simulink model "AFO_Assistance"  (R2024a)
settings: Solver=FixedStepAuto  StartTime=0.0  StopTime=inf  FixedStep=0.001  RelTol=1e-3  EnableMultiTasking=on
libraries: slrealtimeethercatlib x15, simulink_extras x5, simulink x1, slpidlib x1
(part 1 of 2)
settings Model: SimulationMode=external  ExtModeEnableFloating=off  Creator=mbout  LastModifiedBy=Andy
settings SolverCC: ConcurrentTasks=on  AlgebraicLoopSolver=TrustRegion  PositivePriorityOrder=on  AutoInsertRateTranBlk=on  InsertRTBMode=Never (minimum delay)
settings DataIOCC: SaveFormat=Array  SaveState=on  SignalLoggingName=logsOut
settings OptimizationCC: BlockReduction=off  BooleanDataType=off  OptimizeBlockIOStorage=off  BufferReuse=off  ReuseModelBlockBuffer=off  GlobalBufferReuse=off  ExpressionFolding=off  LocalBlockOutputs=off  InitFltsAndDblsToZero=on  OptimizeDataStoreBuffers=off  BusAssignmentInplaceUpdate=off
settings DebuggingCC: SaveWithParameterizedLinksMsg=none  UnderspecifiedInitializationDetection=Classic  MergeDetectMultiDrivingBlocksExec=none  CheckExecutionContextPreStartOutputMsg=on  SignalResolutionControl=TryResolveAllWithWarning  TasksWithSamePriorityMsg=none  ParameterPrecisionLossMsg=none  UnconnectedInputMsg=warning  UnconnectedOutputMsg=warning  UnconnectedLineMsg=warning  SFUnexpectedBacktrackingDiag=warning  SFNoUnconditionalDefaultTransitionDiag=warning  SFExecutionAtInitializationDiag=none  ArithmeticOperatorsInVariantConditions=warning
settings HardwareCC: ProdBitPerLong=64  ProdLongLongMode=on  ProdHWDeviceType=Intel->x86-64 (Linux 64)
settings ModelReferenceCC: EnableRefExpFcnMdlSchedulingChecks=on  PropagateSignalLabelsOutOfModel=off
settings SFSimCC: SimUseLocalCustomCode=off  SimTargetLang=C++
settings RTWCC: Description=Speedgoat Real-Time Target Machine  SystemTargetFile=speedgoat.tlc  TemplateMakefile=slrealtime_default_tmf  RTWUseLocalCustomCode=off  Toolchain=Simulink Real-Time Toolchain  BuildConfiguration=Faster Runs  CodeExecutionProfiling=on  TargetLang=C++  GPUComputeCapability=3.5  DLArmComputeVersion=19.05
settings CodeAppCC: StateflowObjectComments=on
settings SimulinkRealTimeTargetCC: InstructionSetFMA=off  LogToMDFFile=off
settings ConfigComp: CovMetricSettings=dw  CovSaveCumulativeToWorkspaceVar=on  CovSaveSingleToWorkspaceVar=on  CovExternalEMLEnable=off  CovSFcnEnable=off

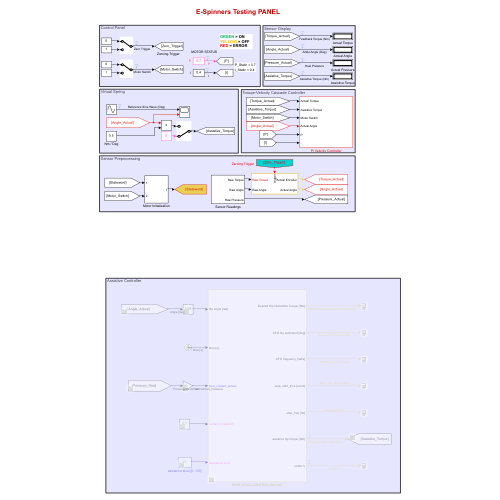
[thumbnail: Simulink's stored preview of the top-level diagram]
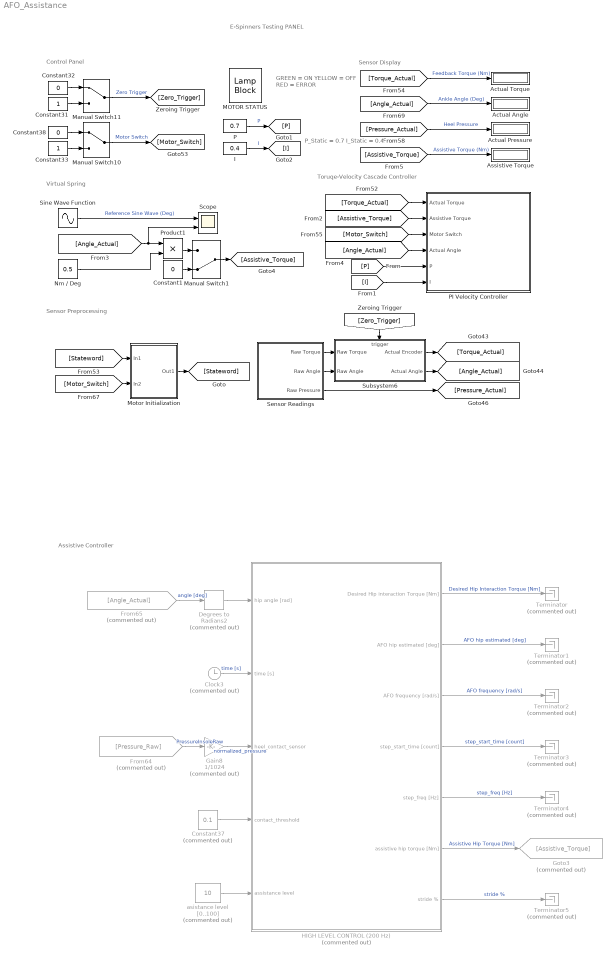
== system AFO_Assistance ==
  note: Sensor Display
  note: E-Spinners Testing PANEL
  note: GREEN = ON
      | YELLOW = OFF
      | RED = ERROR
  note: Control Panel
  note: Toruqe-Velocity Cascade Controller
  note: Sensor Preprocessing
  note: P_Static = 0.7
      | I_Static = 0.4
  note: Assistive Controller
  note: Virtual Spring
  Actual Angle : Display
  Actual Pressure : Display
  Actual Torque : Display
  Assistive Torque : Display
  Clock3 : Clock  Commented=on
  Constant1 : Constant  Value=0
  Constant31 : Constant
  Constant32 : Constant  Value=0
  Constant33 : Constant
  Constant37 : Constant  Commented=on  Value=0.1
  Constant38 : Constant  Value=0
  Degrees to Radians2 : simulink_extras/Transformations/Degrees to Radians  Commented=on
  From64 : From  Commented=on  GotoTag=Pressure_Raw
  From65 : From  Commented=on  GotoTag=Angle_Actual
  Gain8 : Gain  Commented=on  Gain=1/1024
  Goto3 : Goto  Commented=on  GotoTag=Assistive_Torque
  HIGH LEVEL CONTROL (200 Hz) : Subsystem  Commented=on
  I : Constant  Value=0.4
  MOTOR STATUS : LampBlock  LabelPosition=Hide
  Manual Switch1 : ManualSwitch  CurrentSetting=0
  Manual Switch10 : ManualSwitch
  Manual Switch11 : ManualSwitch
  Motor Initialization : Subsystem
  Nm / Deg : Constant  Value=0.5
  P : Constant  Value=0.7
  PI Velocity Controller : Subsystem
  Product1 : Product
  Scope : Scope  NumInputPorts=2
  Sensor Readings : Subsystem
  Sine Wave Function : Sin  Amplitude=24  Frequency=0.5 * 6.28  SampleTime=0
  Subsystem6 : Subsystem  TreatAsAtomicUnit=on
      settings: PortSchema="{\"entries\":[{\"content\":{\"sides\":[{\"content\":{\"connectorIds\":[\"In1\",\"In2\"]},\"type\":\"ConnectorPlacement.EquallySpacedRectSide\",\"uuid\":\"9f3d9f1a-9a54-41ee-920c-c2d0f371d202\"},{\"content\":{\"connectorIds\":[\"Out1\",\"Out2\"],\"side\":\"RIGHT\"},\"type\":\"ConnectorPlacement.EquallySpacedRectSide\",\"uuid\":\"1f39d886-5c2a-4ad9-bf33-c1da713dba43\"},{\"content\":{\"connectorIds\":[\"In3\"],\"side\":\"TOP\"},\"type\":\"ConnectorPlacement.EquallySpacedRectSide\",\"uuid\":\"f96becb7-64eb-4482-a661-ce8cddc3e5ff\"}]},\"type\":\"ConnectorPlacement.EquallySpacedConnector\",\"uuid\":\"ca43ddc1-706b-467a-b9cf-4d299dd568f6\"}],\"packageUris\":[\"http://schema.mathworks.com/mf0/Connector/R2020b\"],\"version\":\"1.0\"}"
  Terminator{,1..5} (6 alike) : Terminator  Commented=on
  asistance level [0..100] : Constant  Commented=on  Value=10  OutMin=[0]  OutMax=[100]  SampleTime=0.01
  wires:
  [Torque_Actual] -> Actual Torque/1  "Feedback Torque (Nm)"
  [Angle_Actual] -> Actual Angle/1  "Ankle Angle (Deg)"
  [Zero_Trigger] -> Subsystem6/3(trigger)
  Subsystem6/2(Actual Angle) -> [Angle_Actual]
  HIGH LEVEL CONTROL (200 Hz)/4(step_start_time [count]) -> Terminator3/1  "step_start_time [count]"
  HIGH LEVEL CONTROL (200 Hz)/7(stride %) -> Terminator5/1  "stride %"
  HIGH LEVEL CONTROL (200 Hz)/3(AFO frequency [rad/s]) -> Terminator2/1  "AFO frequency [rad/s]"
  From64/1 -> Gain8/1  "PressureInsoleRaw"
  Constant32/1 -> Manual Switch11/1
  Subsystem6/1(Actual Encoder) -> [Torque_Actual]
  Degrees to Radians2/1 -> HIGH LEVEL CONTROL (200 Hz)/1(hip angle [rad])
  [Pressure_Actual] -> Actual Pressure/1  "Heel Pressure"
  Gain8/1 -> HIGH LEVEL CONTROL (200 Hz)/3(heel_contact_sensor)  "normalized_pressure"
  HIGH LEVEL CONTROL (200 Hz)/2(AFO hip estimated [deg]) -> Terminator1/1  "AFO hip estimated [deg]"
  From65/1 -> Degrees to Radians2/1  "angle [deg]"
  [Torque_Actual] -> PI Velocity Controller/1(Actual Torque)
  HIGH LEVEL CONTROL (200 Hz)/1(Desired Hip interaction Torque [Nm]) -> Terminator/1  "Desired Hip Interaction Torque [Nm]"
  [I] -> PI Velocity Controller/6(I)
  Constant37/1 -> HIGH LEVEL CONTROL (200 Hz)/4(contact_threshold)
  Constant31/1 -> Manual Switch11/2
  Constant33/1 -> Manual Switch10/2
  [Motor_Switch] -> PI Velocity Controller/3(Motor Switch)
  Constant38/1 -> Manual Switch10/1
  Manual Switch10/1 -> [Motor_Switch]  "Motor Switch"
  [P] -> PI Velocity Controller/5(P)
  Sensor Readings/2(Raw Angle) -> Subsystem6/2(Raw Angle)
  Manual Switch11/1 -> [Zero_Trigger]  "Zero Trigger"
  HIGH LEVEL CONTROL (200 Hz)/6(assistive hip torque [Nm]) -> Goto3/1  "Assistive Hip Torque [Nm]"
  Clock3/1 -> HIGH LEVEL CONTROL (200 Hz)/2(time [s])  "time [s]"
  HIGH LEVEL CONTROL (200 Hz)/5(step_freq [Hz]) -> Terminator4/1  "step_freq [Hz]"
  P/1 -> [P]  "P"
  I/1 -> [I]  "I"
  [Assistive_Torque] -> PI Velocity Controller/2(Assistive Torque)
  [Angle_Actual] -> Product1/1, Scope/2
  Nm / Deg/1 -> Product1/2
  Sine Wave Function/1 -> Scope/1  "Reference Sine Wave (Deg)"
  Manual Switch1/1 -> [Assistive_Torque]
  asistance level [0..100]/1 -> HIGH LEVEL CONTROL (200 Hz)/5(assistance level)
  [Stateword] -> Motor Initialization/1(In1)
  [Motor_Switch] -> Motor Initialization/2(In2)
  Motor Initialization/1(Out1) -> [Stateword]
  Product1/1 -> Manual Switch1/1
  Constant1/1 -> Manual Switch1/2
  [Angle_Actual] -> PI Velocity Controller/4(Actual Angle)
  Sensor Readings/3(Raw Pressure) -> [Pressure_Actual]
  Sensor Readings/1(Raw Torque) -> Subsystem6/1(Raw Torque)
  [Assistive_Torque] -> Assistive Torque/1  "Assistive Torque (Nm)"

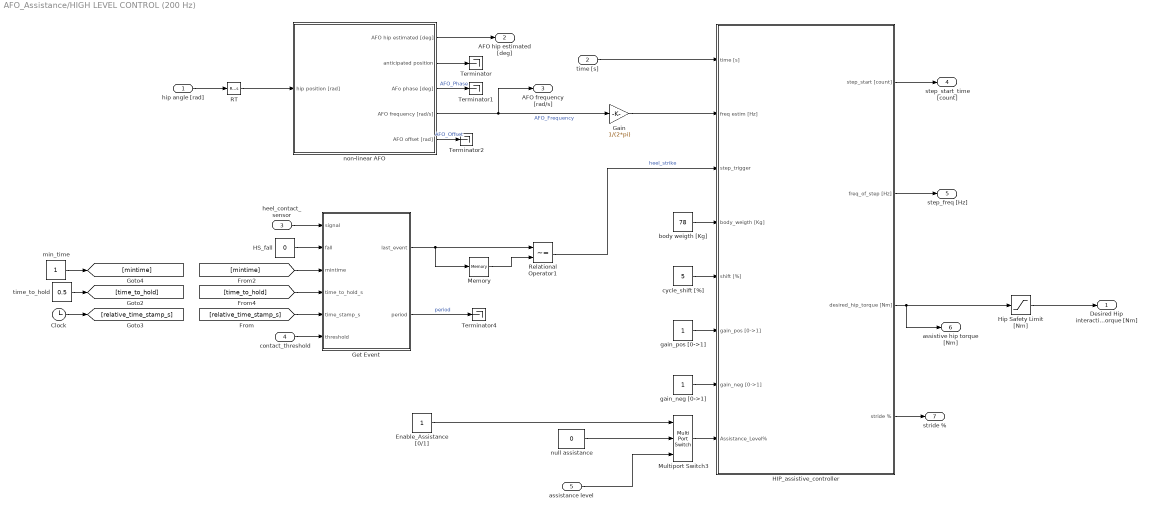
== system AFO_Assistance/HIGH LEVEL CONTROL (200 Hz) ==
  hip angle [rad] : Inport
  time [s] : Inport  Port=2
  heel_contact_sensor : Inport  Port=3
  contact_threshold : Inport  Port=4
  assistance level : Inport  Port=5
  Clock : Clock
  Enable_Assistance [0/1] : Constant  OutMin=[0]  OutMax=[1]  SampleTime=0.01
  Gain : Gain  Gain=1/(2*pi)
  Get Event : Subsystem  TreatAsAtomicUnit=on  SystemSampleTime=1/200
  HIP_assistive_controller : Subsystem
  HS_fall : Constant  Value=0
  Hip Safety Limit [Nm] : Saturate  UpperLimit=50  LowerLimit=-50  SampleTime=0.01
  Memory : Memory
  Multiport Switch3 : MultiPortSwitch  DataPortOrder=Zero-based contiguous  Inputs=2  zeroidx=on  SampleTime=0.01  SaturateOnIntegerOverflow=off  InputSameDT=off
  RT : RateTransition  Deterministic=off  OutPortSampleTime=1/200
  Relational Operator1 : RelationalOperator  Operator=~=  OutDataTypeStr=boolean  RndMeth=Simplest  InputSameDT=off
  Terminator{,1..2,4} (4 alike) : Terminator
  body weigth [Kg] : Constant  Value=78  OutMin=[0]  OutMax=[100]  SampleTime=0.01
  cycle_shift [%] : Constant  Value=5  OutMin=[0]  OutMax=[20]  SampleTime=0.01
  gain_neg [0->1] : Constant  OutMin=[0]  OutMax=[1]  SampleTime=0.01
  gain_pos [0->1] : Constant  OutMin=[0]  OutMax=[1]  SampleTime=0.01
  min_time : Constant
  non-linear AFO : Subsystem
  null assistance : Constant  Value=0  OutMin=[0]  OutMax=[1]  SampleTime=0.01
  time_to_hold : Constant  Value=0.5
  Desired Hip interaction Torque [Nm] : Outport
  AFO hip estimated [deg] : Outport  Port=2
  AFO frequency [rad/s] : Outport  Port=3
  step_start_time [count] : Outport  Port=4
  step_freq [Hz] : Outport  Port=5
  assistive hip torque [Nm] : Outport  Port=6
  stride % : Outport  Port=7
  wires:
  hip angle [rad]/1 -> RT/1
  Hip Safety Limit [Nm]/1 -> Desired Hip interaction Torque [Nm]/1
  non-linear AFO/1(AFO hip estimated [deg]) -> AFO hip estimated [deg]/1
  non-linear AFO/4(AFO frequency [rad/s]) -> Gain/1, AFO frequency [rad/s]/1  "AFO_Frequency"
  Gain/1 -> HIP_assistive_controller/2(freq estim [Hz])
  time [s]/1 -> HIP_assistive_controller/1(time [s])
  HIP_assistive_controller/1(step_start [count]) -> step_start_time [count]/1
  HIP_assistive_controller/2(freq_of_step [Hz]) -> step_freq [Hz]/1
  HIP_assistive_controller/3(desired_hip_torque [Nm]) -> Hip Safety Limit [Nm]/1, assistive hip torque [Nm]/1
  HIP_assistive_controller/4(stride %) -> stride %/1
  body weigth [Kg]/1 -> HIP_assistive_controller/4(body_weigth [Kg])
  cycle_shift [%]/1 -> HIP_assistive_controller/5(shift [%])
  gain_neg [0->1]/1 -> HIP_assistive_controller/7(gain_neg [0->1])
  Enable_Assistance [0/1]/1 -> Multiport Switch3/1
  null assistance/1 -> Multiport Switch3/2
  non-linear AFO/2(anticipated position) -> Terminator/1
  non-linear AFO/3(AFo phase [deg]) -> Terminator1/1  "AFO_Phase"
  non-linear AFO/5(AFO offset [rad]) -> Terminator2/1  "AFO_Offset"
  gain_pos [0->1]/1 -> HIP_assistive_controller/6(gain_pos [0->1])
  Multiport Switch3/1 -> HIP_assistive_controller/8(Assistance_Level%)
  assistance level/1 -> Multiport Switch3/3
  HS_fall/1 -> Get Event/2(fall)
  Relational Operator1/1 -> HIP_assistive_controller/3(step_trigger)  "heel_strike"
  Memory/1 -> Relational Operator1/2
  Get Event/1(last_event) -> Memory/1, Relational Operator1/1
  Get Event/2(period) -> Terminator4/1  "period"
  min_time/1 -> [mintime]
  Clock/1 -> [relative_time_stamp_s]
  contact_threshold/1 -> Get Event/6(threshold)
  [time_to_hold] -> Get Event/4(time_to_hold_s)
  [mintime] -> Get Event/3(mintime)
  [relative_time_stamp_s] -> Get Event/5(time_stamp_s)
  time_to_hold/1 -> [time_to_hold]
  heel_contact_sensor/1 -> Get Event/1(signal)
  RT/1 -> non-linear AFO/1(hip position [rad])

== system AFO_Assistance/Motor Initialization ==
  note: Current Limit in mA
  note: The EtherCAT network initilization and some critical PDO transmissions happen here
  note: Motor Initilization automaticly sends the required command words to the motor to start it from a PRE-OP or Fault state to the Operational State
      | THIS DOES NOT CLEAR ALL POTENTIAL DRIVE ERRORS, JUST THE MOST COMMON ONES
  In1 : Inport
  In2 : Inport  Port=2
  Constant30 : Constant  Value=999
  EtherCAT Initialization Subsystem1 : Subsystem
  Motor Initliazation1 : Stateflow chart  TreatAsAtomicUnit=on  SystemSampleTime=1/100
  Switch4 : Switch  Criteria=u2 > Threshold  SaturateOnIntegerOverflow=off  InputSameDT=off
  Out1 : Outport
  wires:
  In1/1 -> Switch4/1
  EtherCAT Initialization Subsystem1/1(Stateword) -> Out1/1  "StateWord"
  Switch4/1 -> Motor Initliazation1/1(Stateword)
  Motor Initliazation1/1(Motor_controlword) -> EtherCAT Initialization Subsystem1/1(Control Word)  "ControlWord"
  In2/1 -> Switch4/2
  Constant30/1 -> Switch4/3

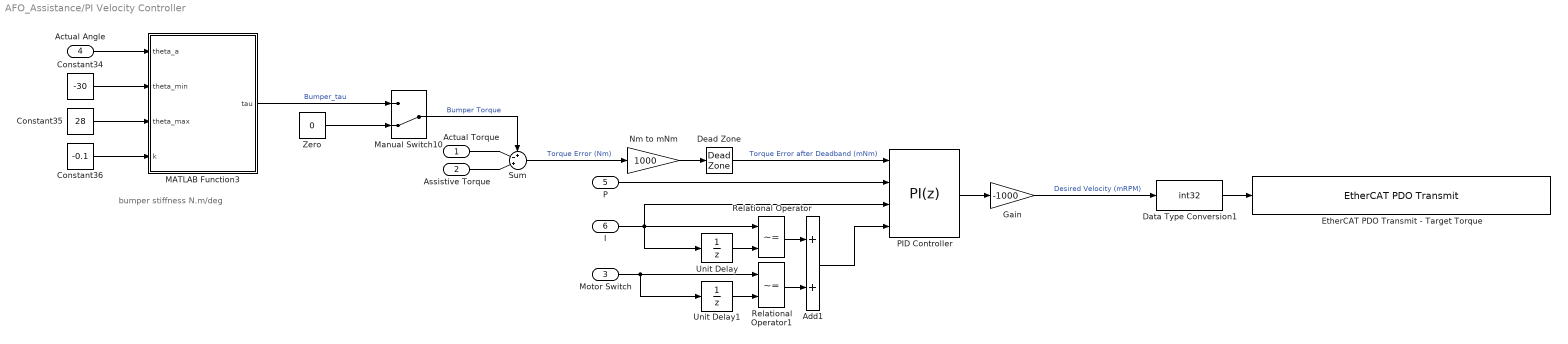
== system AFO_Assistance/PI Velocity Controller ==
  note: bumper stiffness N.m/deg
  Actual Torque : Inport
  Assistive Torque : Inport  Port=2
  Motor Switch : Inport  Port=3
  Actual Angle : Inport  Port=4
  P : Inport  Port=5
  I : Inport  Port=6
  Add1 : Sum
  Constant34 : Constant  Value=-30
  Constant35 : Constant  Value=28
  Constant36 : Constant  Value=-0.1
  Data Type Conversion1 : DataTypeConversion  OutDataTypeStr=int32  SaturateOnIntegerOverflow=off  RndMeth=Floor
  Dead Zone : DeadZone  LowerValue=0  UpperValue=0
  EtherCAT PDO Transmit - Target Torque : slrealtimeethercatlib/EtherCAT PDO Transmit  Priority=3  sig_name=Drive 1 (AMC Servo Drive).Outputs.Target Velocity  sig_offset=328  sig_type=int32  type_size=32  sig_dim=1  device_id=0  sample_time=0.001000
  Gain : Gain  Gain=-1000
  MATLAB Function3 : MATLAB Function  TreatAsAtomicUnit=on
  Manual Switch10 : ManualSwitch  CurrentSetting=0
  Nm to mNm : Gain  Gain=1000
  PID Controller : slpidlib/PID Controller  Controller=PI  Form=Parallel  TimeDomain=Discrete-time  UseExternalTs=off  SampleTime=-1  IntegratorMethod=Forward Euler  FilterMethod=Forward Euler  ControllerParametersSource=external  P=1  I=1  UseKiTs=off  D=0  UseExternalDerivativeSource=off  N=100  UseFilter=on  TunerSelectOption=Transfer Function Based (PID Tuner App)  InitialConditionSource=internal  InitialConditionForIntegrator=0  InitialConditionForFilter=0  DifferentiatorICPrevScaledInput=0  ExternalReset=either  TrackingMode=off  Kt=1  LimitOutput=on  SatLimitsSource=internal  UpperSaturationLimit=5000  LowerSaturationLimit=-5000  LinearizeAsGain=on  AntiWindupMode=none  Kb=1  LimitIntegrator=off  UpperIntegratorSaturationLimit=inf  LowerIntegratorSaturationLimit=-inf  POutMin=[]  POutMax=[]  IOutMin=[]  IOutMax=[]  DOutMin=[]  DOutMax=[]  NOutMin=[]  NOutMax=[]  SumOutMin=[]  SumOutMax=[]  SaturationOutMin=[]  SaturationOutMax=[]  PParamMin=[]  PParamMax=[]  IParamMin=[]  IParamMax=[]  DParamMin=[]  DParamMax=[]  NParamMin=[]  NParamMax=[]  KbParamMin=[]  KbParamMax=[]  KtParamMin=[]  KtParamMax=[]  KbOutMin=[]  KbOutMax=[]  KtOutMin=[]  KtOutMax=[]  IntegratorOutMin=[]  IntegratorOutMax=[]  FilterOutMin=[]  FilterOutMax=[]  SumI1OutMin=[]  SumI1OutMax=[]  SumI2OutMin=[]  SumI2OutMax=[]  SumI3OutMin=[]  SumI3OutMax=[]  SumI4OutMin=[]  SumI4OutMax=[]  SumDOutMin=[]  SumDOutMax=[]  DifferentiatorOutMin=[]  DifferentiatorOutMax=[]  FilterDiffOutCoefMin=[]  FilterDiffOutCoefMax=[]  ReciprocalOutMin=[]  ReciprocalOutMax=[]  SumDenOutMin=[]  SumDenOutMax=[]  SumNumOutMin=[]  SumNumOutMax=[]  DivideOutMin=[]  DivideOutMax=[]  UdiffTsProdOutMin=[]  UdiffTsProdOutMax=[]  NTsProdOutMin=[]  NTsProdOutMax=[]  UintegralTsProdOutMin=[]  UintegralTsProdOutMax=[]  UngainTsProdOutMin=[]  UngainTsProdOutMax=[]  ClampingZeroOutDataTypeStr=Inherit: Inherit via back propagation  ClampingZeroOutMin=[]  ClampingZeroOutMax=[]  FilterDenConstantOutDataTypeStr=Inherit: Inherit via back propagation  FilterDenConstantOutMin=[]  FilterDenConstantOutMax=[]  PCopyOutDataTypeStr=Inherit: Inherit via back propagation  PCopyOutMin=[]  PCopyOutMax=[]  NCopyOutDataTypeStr=Inherit: Inherit via back propagation  NCopyOutMin=[]  NCopyOutMax=[]  IntegratorContinuousStateAttributes=''  IntegratorStateMustResolveToSignalObject=off  IntegratorRTWStateStorageClass=Auto  FilterContinuousStateAttributes=''  FilterStateMustResolveToSignalObject=off  FilterRTWStateStorageClass=Auto  ParallelPVariant=ExternalParameters  IdealPVariant=Disabled  IVariant=ExternalParameters  DVariant=Disabled  IntegratorVariant=Discrete  SatVariant=Enabled  AWVariant=Passthrough  PCopyVariant=Disabled  TRVariant=Disabled  FdbkBlocksVariant=Forward  IdealPFdbkVariant=Disabled  SatFdbkVariant=Disabled  DerivativeFilterVariant=Disabled  NVariant=Disabled  NCopyVariant=Disabled_SignalSpec  FilterICVariant=Disabled  IntegratorICVariant=InternalICs  ExternalResetVariant=ExternalReset  TRSumVariant=Passthrough  SumFdbkVariant=Disabled  SumVariant=Sum_PI  TsampFilterVariant=InternalTs  TsampNgainVariant=Passthrough  TsampIntegralVariant=Disabled_SignalSpec  ExternalSaturationOutDataTypeStr=Inherit: Same as second input  DerivativeSourceVariant=Disabled
  Relational Operator : RelationalOperator  Operator=~=  OutDataTypeStr=boolean  RndMeth=Simplest  InputSameDT=off
  Relational Operator1 : RelationalOperator  Operator=~=  OutDataTypeStr=boolean  RndMeth=Simplest  InputSameDT=off
  Sum : Sum  Inputs=+-+|
  Unit Delay : UnitDelay  SampleTime=-1  HasFrameUpgradeWarning=on
  Unit Delay1 : UnitDelay  SampleTime=-1  HasFrameUpgradeWarning=on
  Zero : Constant  Value=0
  wires:
  P/1 -> PID Controller/2
  Data Type Conversion1/1 -> EtherCAT PDO Transmit - Target Torque/1
  Motor Switch/1 -> Unit Delay1/1, Relational Operator1/1
  Dead Zone/1 -> PID Controller/1  "Torque Error after Deadband (mNm)"
  Unit Delay/1 -> Relational Operator/2
  I/1 -> Unit Delay/1, PID Controller/3, Relational Operator/1
  Zero/1 -> Manual Switch10/2
  Unit Delay1/1 -> Relational Operator1/2
  Relational Operator/1 -> Add1/1
  Relational Operator1/1 -> Add1/2
  Manual Switch10/1 -> Sum/1  "Bumper Torque"
  Assistive Torque/1 -> Sum/3
  Gain/1 -> Data Type Conversion1/1  "Desired Velocity (mRPM)"
  Actual Torque/1 -> Sum/2
  Sum/1 -> Nm to mNm/1  "Torque Error (Nm)"
  PID Controller/1 -> Gain/1
  Add1/1 -> PID Controller/4
  Nm to mNm/1 -> Dead Zone/1
  Actual Angle/1 -> MATLAB Function3/1(theta_a)
  MATLAB Function3/1(tau) -> Manual Switch10/1  "Bumper_tau"
  Constant35/1 -> MATLAB Function3/3(theta_max)
  Constant34/1 -> MATLAB Function3/2(theta_min)
  Constant36/1 -> MATLAB Function3/4(k)

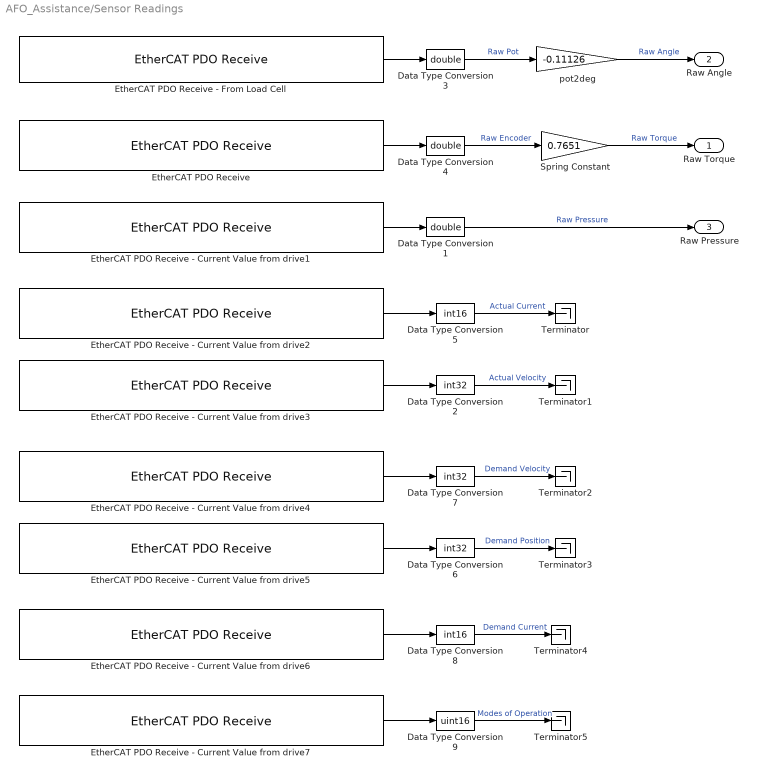
== system AFO_Assistance/Sensor Readings ==
  Data Type Conversion1 : DataTypeConversion  OutDataTypeStr=double  SaturateOnIntegerOverflow=off  RndMeth=Floor
  Data Type Conversion2 : DataTypeConversion  OutDataTypeStr=int32  SaturateOnIntegerOverflow=off  RndMeth=Floor
  Data Type Conversion3 : DataTypeConversion  OutDataTypeStr=double  SaturateOnIntegerOverflow=off  RndMeth=Floor
  Data Type Conversion4 : DataTypeConversion  OutDataTypeStr=double  SaturateOnIntegerOverflow=off  RndMeth=Floor
  Data Type Conversion5 : DataTypeConversion  OutDataTypeStr=int16  SaturateOnIntegerOverflow=off  RndMeth=Floor
  Data Type Conversion6 : DataTypeConversion  OutDataTypeStr=int32  SaturateOnIntegerOverflow=off  RndMeth=Floor
  Data Type Conversion7 : DataTypeConversion  OutDataTypeStr=int32  SaturateOnIntegerOverflow=off  RndMeth=Floor
  Data Type Conversion8 : DataTypeConversion  OutDataTypeStr=int16  SaturateOnIntegerOverflow=off  RndMeth=Floor
  Data Type Conversion9 : DataTypeConversion  OutDataTypeStr=uint16  SaturateOnIntegerOverflow=off  RndMeth=Floor
  EtherCAT PDO Receive : slrealtimeethercatlib/EtherCAT PDO Receive  Priority=2  sig_name=Box 2 (teensySensoryMB).Inputs.Force2  sig_offset=680  sig_type=double  type_size=64  sig_dim=1  device_id=0  sample_time=0.001000
  EtherCAT PDO Receive - Current Value from drive1 : slrealtimeethercatlib/EtherCAT PDO Receive  Priority=2  sig_name=Box 2 (teensySensoryMB).Inputs.Force3  sig_offset=744  sig_type=double  type_size=64  sig_dim=1  device_id=0  sample_time=0.001000
  EtherCAT PDO Receive - Current Value from drive2 : slrealtimeethercatlib/EtherCAT PDO Receive  Priority=2  sig_name=Drive 1 (AMC Servo Drive).Inputs.Actual Current  sig_offset=392  sig_type=int16  type_size=16  sig_dim=1  device_id=0  sample_time=0.001000
  EtherCAT PDO Receive - Current Value from drive3 : slrealtimeethercatlib/EtherCAT PDO Receive  Priority=2  sig_name=Drive 1 (AMC Servo Drive).Inputs.Actual Velocity  sig_offset=360  sig_type=int32  type_size=32  sig_dim=1  device_id=0  sample_time=0.001000
  EtherCAT PDO Receive - Current Value from drive4 : slrealtimeethercatlib/EtherCAT PDO Receive  Priority=2  sig_name=Drive 1 (AMC Servo Drive).Inputs.Velocity Demand  sig_offset=408  sig_type=int32  type_size=32  sig_dim=1  device_id=0  sample_time=0.001000
  EtherCAT PDO Receive - Current Value from drive5 : slrealtimeethercatlib/EtherCAT PDO Receive  Priority=2  sig_name=Drive 1 (AMC Servo Drive).Inputs.Position Demand  sig_offset=440  sig_type=int32  type_size=32  sig_dim=1  device_id=0  sample_time=0.001000
  EtherCAT PDO Receive - Current Value from drive6 : slrealtimeethercatlib/EtherCAT PDO Receive  Priority=2  sig_name=Drive 1 (AMC Servo Drive).Inputs.Iq - Demand  sig_offset=504  sig_type=uint16  type_size=16  sig_dim=1  device_id=0  sample_time=0.001000
  EtherCAT PDO Receive - Current Value from drive7 : slrealtimeethercatlib/EtherCAT PDO Receive  Priority=2  sig_name=Drive 1 (AMC Servo Drive).Inputs.Modes of Operation Display  sig_offset=472  sig_type=uint16  type_size=16  sig_dim=1  device_id=0  sample_time=0.001000
  EtherCAT PDO Receive - From Load Cell : slrealtimeethercatlib/EtherCAT PDO Receive  Priority=2  sig_name=Box 2 (teensySensoryMB).Inputs.Force1  sig_offset=616  sig_type=double  type_size=64  sig_dim=1  device_id=0  sample_time=0.001000
  Spring Constant : Gain  Gain=0.7651
  Terminator{,1..5} (6 alike) : Terminator
  pot2deg : Gain  Gain=-0.11126
  Raw Torque : Outport
  Raw Angle : Outport  Port=2
  Raw Pressure : Outport  Port=3
  wires:
  pot2deg/1 -> Raw Angle/1  "Raw Angle"
  EtherCAT PDO Receive - From Load Cell/1 -> Data Type Conversion3/1
  EtherCAT PDO Receive - Current Value from drive1/1 -> Data Type Conversion1/1
  Data Type Conversion3/1 -> pot2deg/1  "Raw Pot"
  EtherCAT PDO Receive/1 -> Data Type Conversion4/1
  Data Type Conversion1/1 -> Raw Pressure/1  "Raw Pressure"
  Data Type Conversion5/1 -> Terminator/1  "Actual Current"
  EtherCAT PDO Receive - Current Value from drive2/1 -> Data Type Conversion5/1
  EtherCAT PDO Receive - Current Value from drive3/1 -> Data Type Conversion2/1
  Data Type Conversion2/1 -> Terminator1/1  "Actual Velocity"
  Data Type Conversion6/1 -> Terminator3/1  "Demand Position"
  EtherCAT PDO Receive - Current Value from drive4/1 -> Data Type Conversion7/1
  EtherCAT PDO Receive - Current Value from drive5/1 -> Data Type Conversion6/1
  Data Type Conversion7/1 -> Terminator2/1  "Demand Velocity"
  EtherCAT PDO Receive - Current Value from drive6/1 -> Data Type Conversion8/1
  Data Type Conversion8/1 -> Terminator4/1  "Demand Current"
  Data Type Conversion9/1 -> Terminator5/1  "Modes of Operation"
  EtherCAT PDO Receive - Current Value from drive7/1 -> Data Type Conversion9/1
  Data Type Conversion4/1 -> Spring Constant/1  "Raw Encoder"
  Spring Constant/1 -> Raw Torque/1  "Raw Torque"

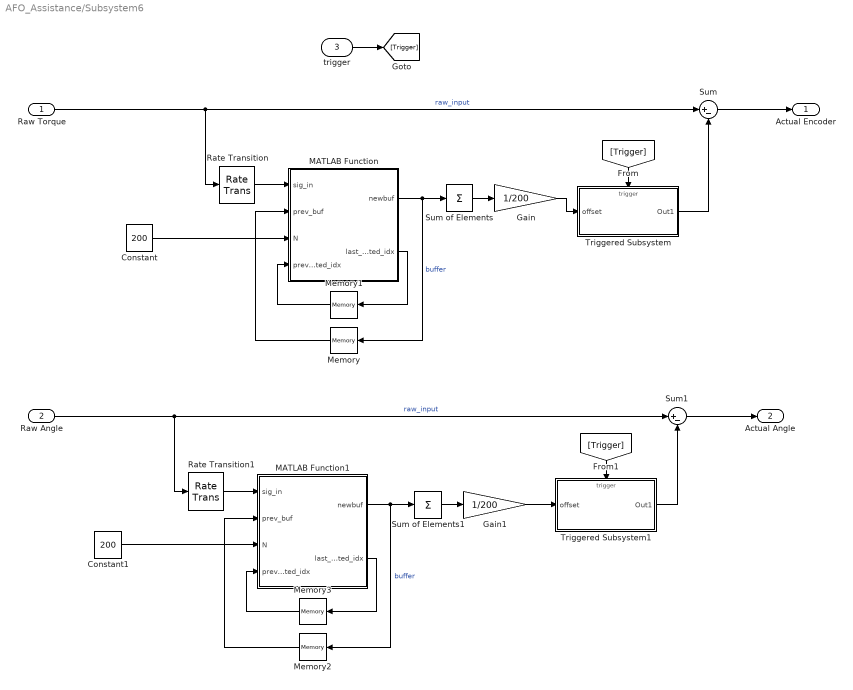
== system AFO_Assistance/Subsystem6 ==
  Raw Torque : Inport
  Raw Angle : Inport  Port=2
  trigger : Inport  Port=3
  Constant : Constant  Value=200
  Constant1 : Constant  Value=200
  Gain : Gain  Gain=1/200
  Gain1 : Gain  Gain=1/200
  MATLAB Function : MATLAB Function  TreatAsAtomicUnit=on  SystemSampleTime=1/200
  MATLAB Function1 : MATLAB Function  TreatAsAtomicUnit=on  SystemSampleTime=1/200
  Memory : Memory  InitialCondition=zeros(200,1)
  Memory1 : Memory
  Memory2 : Memory  InitialCondition=zeros(200,1)
  Memory3 : Memory
  Rate Transition : RateTransition  OutPortSampleTime=1/200
  Rate Transition1 : RateTransition  OutPortSampleTime=1/200
  Sum : Sum  Inputs=|+-
  Sum of Elements : Sum  Inputs=+
  Sum of Elements1 : Sum  Inputs=+
  Sum1 : Sum  Inputs=|+-
  Triggered Subsystem : Subsystem  TreatAsAtomicUnit=on
  Triggered Subsystem1 : Subsystem  TreatAsAtomicUnit=on
  Actual Encoder : Outport
  Actual Angle : Outport  Port=2
  wires:
  Rate Transition/1 -> MATLAB Function/1(sig_in)
  Memory1/1 -> MATLAB Function/4(prev_updated_idx)
  MATLAB Function/2(last_updated_idx) -> Memory1/1
  Memory/1 -> MATLAB Function/2(prev_buf)
  Constant/1 -> MATLAB Function/3(N)
  Sum/1 -> Actual Encoder/1
  Sum of Elements/1 -> Gain/1
  Triggered Subsystem/1(Out1) -> Sum/2
  Gain/1 -> Triggered Subsystem/1(offset)
  MATLAB Function/1(newbuf) -> Memory/1, Sum of Elements/1  "buffer"
  Raw Torque/1 -> Sum/1, Rate Transition/1  "raw_input"
  MATLAB Function1/2(last_updated_idx) -> Memory3/1
  [Trigger] -> Triggered Subsystem1/Trigger
  Memory2/1 -> MATLAB Function1/2(prev_buf)
  Gain1/1 -> Triggered Subsystem1/1(offset)
  Triggered Subsystem1/1(Out1) -> Sum1/2
  Sum of Elements1/1 -> Gain1/1
  MATLAB Function1/1(newbuf) -> Memory2/1, Sum of Elements1/1  "buffer"
  Constant1/1 -> MATLAB Function1/3(N)
  Rate Transition1/1 -> MATLAB Function1/1(sig_in)
  Sum1/1 -> Actual Angle/1
  Raw Angle/1 -> Sum1/1, Rate Transition1/1  "raw_input"
  Memory3/1 -> MATLAB Function1/4(prev_updated_idx)
  trigger/1 -> [Trigger]
  [Trigger] -> Triggered Subsystem/Trigger

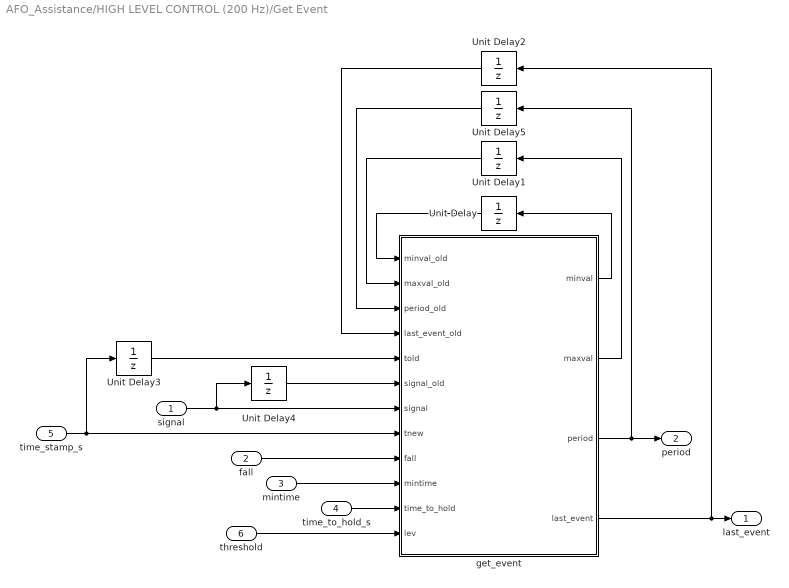
== system AFO_Assistance/HIGH LEVEL CONTROL (200 Hz)/Get Event ==
  signal : Inport
  fall : Inport  Port=2
  mintime : Inport  Port=3
  time_to_hold_s : Inport  Port=4
  time_stamp_s : Inport  Port=5
  threshold : Inport  Port=6
  Unit Delay : UnitDelay  InitialCondition=4.5  SampleTime=-1
  Unit Delay1 : UnitDelay  InitialCondition=0.5  SampleTime=-1
  Unit Delay{2..5} (4 alike) : UnitDelay  SampleTime=-1
  get_event : MATLAB Function  TreatAsAtomicUnit=on
  last_event : Outport
  period : Outport  Port=2
  wires:
  get_event/1(minval) -> Unit Delay/1
  get_event/2(maxval) -> Unit Delay1/1
  get_event/4(last_event) -> Unit Delay2/1, last_event/1
  Unit Delay/1 -> get_event/1(minval_old)
  Unit Delay1/1 -> get_event/2(maxval_old)
  Unit Delay2/1 -> get_event/4(last_event_old)
  time_to_hold_s/1 -> get_event/11(time_to_hold)
  mintime/1 -> get_event/10(mintime)
  fall/1 -> get_event/9(fall)
  Unit Delay3/1 -> get_event/5(told)
  Unit Delay4/1 -> get_event/6(signal_old)
  threshold/1 -> get_event/12(lev)
  get_event/3(period) -> Unit Delay5/1, period/1
  signal/1 -> get_event/7(signal), Unit Delay4/1
  Unit Delay5/1 -> get_event/3(period_old)
  time_stamp_s/1 -> get_event/8(tnew), Unit Delay3/1

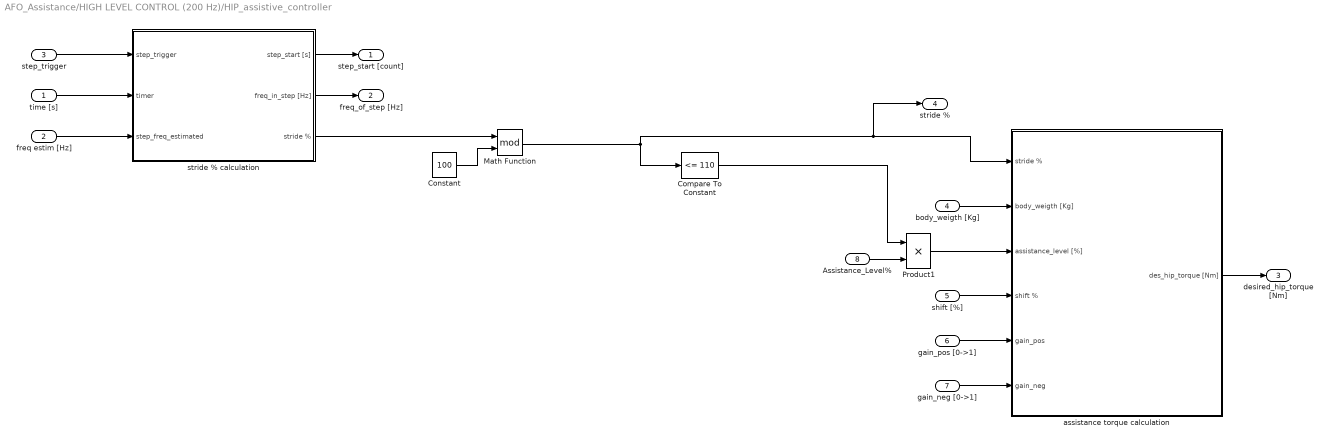
== system AFO_Assistance/HIGH LEVEL CONTROL (200 Hz)/HIP_assistive_controller ==
  time [s] : Inport
  freq estim [Hz] : Inport  Port=2
  step_trigger : Inport  Port=3
  body_weigth [Kg] : Inport  Port=4
  shift [%] : Inport  Port=5
  gain_pos [0->1] : Inport  Port=6
  gain_neg [0->1] : Inport  Port=7
  Assistance_Level% : Inport  Port=8
  Compare To Constant : simulink/Logic and Bit Operations/Compare To Constant  relop=<=  const=110  OutDataTypeStr=uint8
  Constant : Constant  Value=100
  Math Function : Math  Operator=mod
  Product1 : Product  RndMeth=Zero  SampleTime=0.01
  assistance torque calculation : Subsystem
  stride % calculation : Subsystem
  step_start [count] : Outport
  freq_of_step [Hz] : Outport  Port=2
  desired_hip_torque [Nm] : Outport  Port=3
  stride % : Outport  Port=4
  wires:
  body_weigth [Kg]/1 -> assistance torque calculation/2(body_weigth [Kg])
  Math Function/1 -> assistance torque calculation/1(stride %), stride %/1, Compare To Constant/1
  step_trigger/1 -> stride % calculation/1(step_trigger)
  stride % calculation/1(step_start [s]) -> step_start [count]/1
  time [s]/1 -> stride % calculation/2(timer)
  stride % calculation/2(freq_in_step [Hz]) -> freq_of_step [Hz]/1
  freq estim [Hz]/1 -> stride % calculation/3(step_freq_estimated)
  assistance torque calculation/1(des_hip_torque [Nm]) -> desired_hip_torque [Nm]/1
  Compare To Constant/1 -> Product1/1
  shift [%]/1 -> assistance torque calculation/4(shift %)
  gain_pos [0->1]/1 -> assistance torque calculation/5(gain_pos)
  gain_neg [0->1]/1 -> assistance torque calculation/6(gain_neg)
  Product1/1 -> assistance torque calculation/3(assistance_level [%])
  Assistance_Level%/1 -> Product1/2
  stride % calculation/3(stride %) -> Math Function/1
  Constant/1 -> Math Function/2

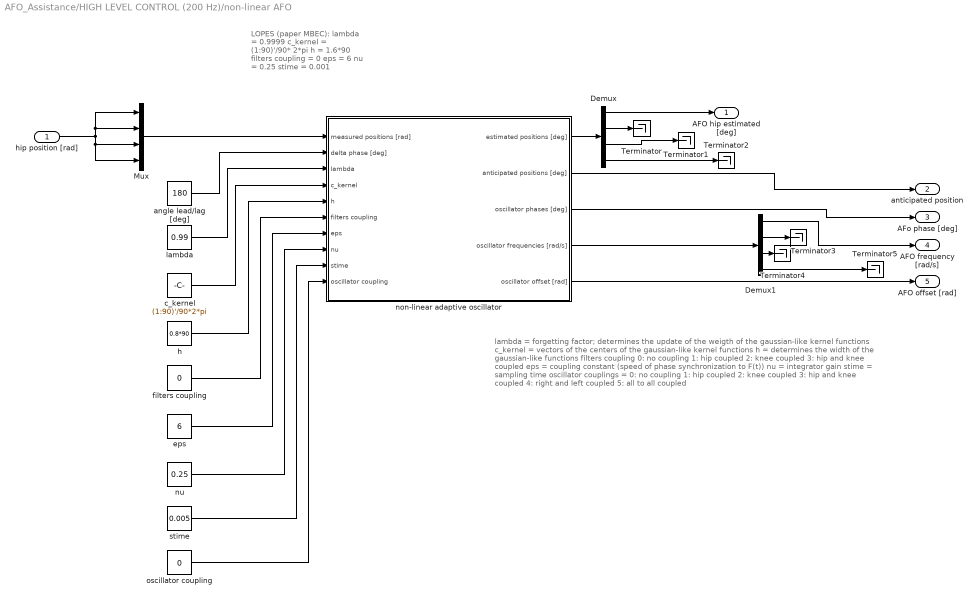
== system AFO_Assistance/HIGH LEVEL CONTROL (200 Hz)/non-linear AFO ==
  note: LOPES (paper MBEC):
      | lambda = 0.9999
      | c_kernel = (1:90)'/90* 2*pi
      | h = 1.6*90
      | filters coupling = 0
      | eps = 6
      | nu = 0.25
      | stime = 0.001
  note: lambda = forgetting factor; determines the update of the weigth of the gaussian-like kernel functions
      | c_kernel = vectors of the centers of the gaussian-like kernel functions
      | h = determines the width of the gaussian-like functions
      | filters coupling
      | 0: no coupling
      | 1: hip coupled
      | 2: knee coupled
      | 3: hip and knee coupled
      | eps = coupling constant (speed of phase synchronization to F(t))
      | nu = integrator gain
      | stime = sampling time
      | oscillator couplings =
      | 0: no coupling
      | 1: hip coupled
      | 2: knee coupled
      | 3: hip and knee coupled
      | 4: right and left coupled
      | 5: all to all coupled
  hip position [rad] : Inport
  Demux : Demux
  Demux1 : Demux
  Mux : Mux
  Terminator{,1..5} (6 alike) : Terminator
  angle lead/lag [deg] : Constant  Value=180  SampleTime=0.01
  c_kernel : Constant  Value=(1:90)'/90*2*pi  SampleTime=0.01
  eps : Constant  Value=6  SampleTime=0.01
  filters coupling : Constant  Value=0  SampleTime=0.01
  h : Constant  Value=0.8*90  SampleTime=0.01
  lambda : Constant  Value=0.99  SampleTime=0.01
  non-linear adaptive oscillator : Subsystem
  nu : Constant  Value=0.25  SampleTime=0.01
  oscillator coupling : Constant  Value=0  SampleTime=0.01
  stime : Constant  Value=0.005  SampleTime=0.01
  AFO hip estimated [deg] : Outport
  anticipated position : Outport  Port=2
  AFo phase [deg] : Outport  Port=3
  AFO frequency [rad/s] : Outport  Port=4
  AFO offset [rad] : Outport  Port=5
  wires:
  angle lead/lag [deg]/1 -> non-linear adaptive oscillator/2(delta phase [deg])
  lambda/1 -> non-linear adaptive oscillator/3(lambda)
  c_kernel/1 -> non-linear adaptive oscillator/4(c_kernel)
  h/1 -> non-linear adaptive oscillator/5(h)
  filters coupling/1 -> non-linear adaptive oscillator/6(filters coupling)
  eps/1 -> non-linear adaptive oscillator/7(eps)
  stime/1 -> non-linear adaptive oscillator/9(stime)
  nu/1 -> non-linear adaptive oscillator/8(nu)
  oscillator coupling/1 -> non-linear adaptive oscillator/10(oscillator coupling)
  Mux/1 -> non-linear adaptive oscillator/1(measured positions [rad])
  non-linear adaptive oscillator/1(estimated positions [deg]) -> Demux/1
  Demux/1 -> AFO hip estimated [deg]/1
  hip position [rad]/1 -> Mux/1, Mux/2, Mux/4, Mux/3
  non-linear adaptive oscillator/2(anticipated positions [deg]) -> anticipated position/1
  non-linear adaptive oscillator/3(oscillator phases [deg]) -> AFo phase [deg]/1
  non-linear adaptive oscillator/5(oscillator offset [rad]) -> AFO offset [rad]/1
  non-linear adaptive oscillator/4(oscillator frequencies [rad/s]) -> Demux1/1
  Demux1/1 -> AFO frequency [rad/s]/1
  Demux/2 -> Terminator/1
  Demux/3 -> Terminator1/1
  Demux/4 -> Terminator2/1
  Demux1/2 -> Terminator3/1
  Demux1/3 -> Terminator4/1
  Demux1/4 -> Terminator5/1

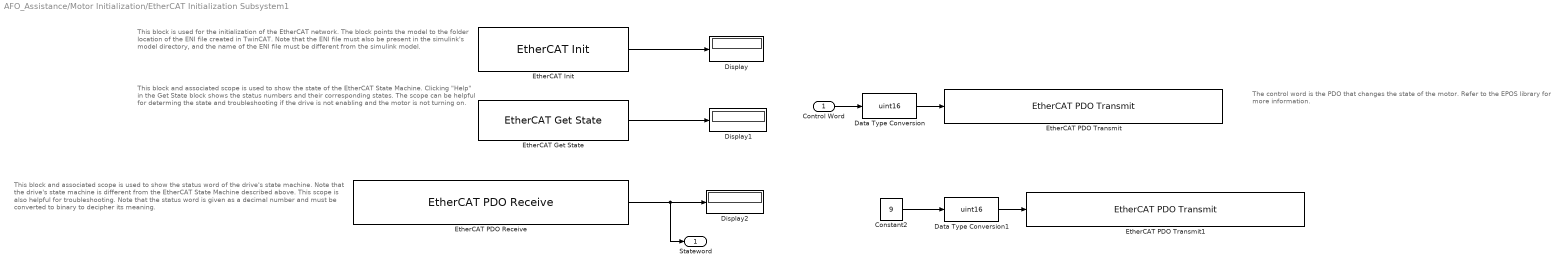
== system AFO_Assistance/Motor Initialization/EtherCAT Initialization Subsystem1 ==
  note: This block is used for the initialization of the EtherCAT network. The block points the model to the folder location of the ENI file created in TwinCAT. Note that the ENI file must also be present in the simulink's model directory, and the name of the ENI file must be different from the simulink model.
  note: This block and associated scope is used to show the state of the EtherCAT State Machine. Clicking "Help" in the Get State block shows the status numbers and their corresponding states. The scope can be helpful for determing the state and troubleshooting if the drive is not enabling and the motor is not turning on.
  note: This block and associated scope is used to show the status word of the drive's state machine. Note that the drive's state machine is different from the EtherCAT State Machine described above. This scope is also helpful for troubleshooting. Note that the status word is given as a decimal number and must be converted to binary to decipher its meaning.
  note: The control word is the PDO that changes the state of the motor. Refer to the EPOS library for more information.
  Control Word : Inport
  Constant2 : Constant  Value=9
  Data Type Conversion : DataTypeConversion  OutDataTypeStr=uint16  SaturateOnIntegerOverflow=off  RndMeth=Floor
  Data Type Conversion1 : DataTypeConversion  OutDataTypeStr=uint16  SaturateOnIntegerOverflow=off  RndMeth=Floor
  Display : Display
      settings: Format=hex (Stored Integer)
  Display1 : Display
  Display2 : Display
  EtherCAT Get State : slrealtimeethercatlib/EtherCAT Get State  device_id=0  sample_time=0
  EtherCAT Init : slrealtimeethercatlib/EtherCAT Init  Priority=0  config_file=C:\Users\Andy\Documents\Ankle-Foot-Orthosis\simulink\hello3_amc.xml  device_id=0  portnum=1  initstate=2  dctuning=2  enaDebug=1  logFile='c:\dbglog.txt'  sample_time=0.001000  DCMode=0
  EtherCAT PDO Receive : slrealtimeethercatlib/EtherCAT PDO Receive  Priority=2  sig_name=Drive 1 (AMC Servo Drive).Inputs.Status Word  sig_offset=312  sig_type=uint16  type_size=16  sig_dim=1  device_id=0  sample_time=0.001000
  EtherCAT PDO Transmit : slrealtimeethercatlib/EtherCAT PDO Transmit  Priority=3  sig_name=Drive 1 (AMC Servo Drive).Outputs.Control Word  sig_offset=312  sig_type=uint16  type_size=16  sig_dim=1  device_id=0  sample_time=0.001000
  EtherCAT PDO Transmit1 : slrealtimeethercatlib/EtherCAT PDO Transmit  Priority=3  sig_name=Drive 1 (AMC Servo Drive).Outputs.Modes of Operation  sig_offset=360  sig_type=uint16  type_size=16  sig_dim=1  device_id=0  sample_time=0.001000
  Stateword : Outport
  wires:
  EtherCAT PDO Receive/1 -> Stateword/1, Display2/1
  EtherCAT Get State/1 -> Display1/1
  EtherCAT Init/1 -> Display/1
  Data Type Conversion/1 -> EtherCAT PDO Transmit/1
  Control Word/1 -> Data Type Conversion/1
  Constant2/1 -> Data Type Conversion1/1
  Data Type Conversion1/1 -> EtherCAT PDO Transmit1/1

== system AFO_Assistance/Subsystem6/Triggered Subsystem ==
  offset : Inport
  Trigger : TriggerPort  VariantControl=(inherit)
  Out1 : Outport
  wires:
  offset/1 -> Out1/1

== system AFO_Assistance/Subsystem6/Triggered Subsystem1 ==
  offset : Inport
  Trigger : TriggerPort  VariantControl=(inherit)
  Out1 : Outport
  wires:
  offset/1 -> Out1/1

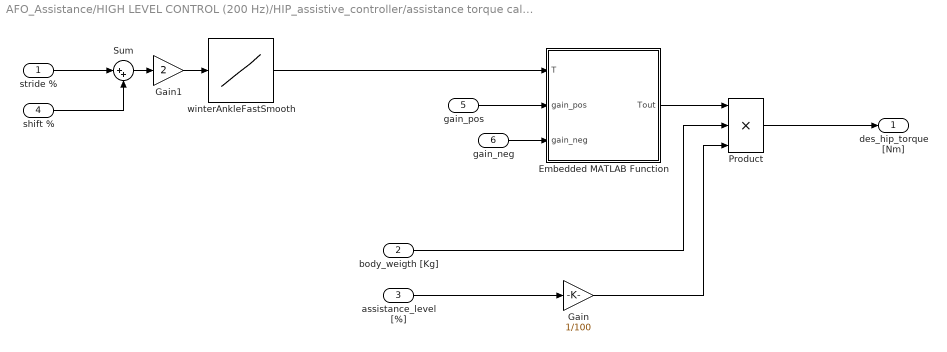
== system AFO_Assistance/HIGH LEVEL CONTROL (200 Hz)/HIP_assistive_controller/assistance torque calculation ==
  stride % : Inport
  body_weigth [Kg] : Inport  Port=2
  assistance_level [%] : Inport  Port=3
  shift % : Inport  Port=4
  gain_pos : Inport  Port=5
  gain_neg : Inport  Port=6
  Embedded MATLAB Function : MATLAB Function  TreatAsAtomicUnit=on
  Gain : Gain  Gain=1/100  SampleTime=0.01
  Gain1 : Gain  Gain=2
  Product : Product  Inputs=3  RndMeth=Zero
  Sum : Sum  Inputs=|++
  winterAnkleFastSmooth : Lookup  InputValues=[0:200]  Table=|  SaturateOnIntegerOverflow=off
      | [-0.00700000000000000
      | -0.00198044104598932
      | -0.00904907548113065
      | -0.0250931721757067
      | -0.0470000000000000
      | -0.0716568278242934
      | -0.0959509245188694
      | -0.116769558954011
      | -0.131000000000000
      | -0.136360997656837
      | -0.133897226443392
      | -0.125484842008251
      | -0.113000000000000
      | -0.0979929315483575
      | -0.0807101697075629
      | -0.0610723230129869
      | -0.0390000000000000
      | -0.0144641511497329
      | 0.0123629052736435
      | 0.0412585090601981
      | 0.0720000000000000
      | 0.104333911147289
      | 0.137883548612989
      | 0.172241411772194
      | 0.207000000000000
      | 0.241722256560577
      | 0.275852900274400
      | 0.308807093851024
      | 0.340000000000000
      | 0.368933312610405
      | 0.395454850289409
      | 0.419498962823709
      | 0.441000000000000
      | 0.459966367997805
      | 0.476702698567963
      | 0.491587679854139
      | 0.505000000000000
      | 0.517248090398375
      | 0.528359355438741
      | 0.538290942759736
      | 0.547000000000000
      | 0.554463145408695
      | 0.560734879677075
      | 0.565889174106917
      | 0.570000000000000
      | 0.573149327966846
      | 0.575451125852960
      | 0.577027360812594
      | 0.578000000000000
      | 0.578502042723923
      | 0.578710616911085
      | 0.578813882642705
      | 0.579000000000000
      | 0.579451876137464
      | 0.580331406502699
      | 0.581795233616584
      | 0.584000000000000
      | 0.587112327726223
      | 0.591338757078120
      | 0.596895807890957
      | 0.604000000000000
      | 0.612880062957646
      | 0.623813565184823
      | 0.637090284819588
      | 0.653000000000000
      | 0.671711170443192
      | 0.692906982182590
      | 0.716149302830693
      | 0.741000000000000
      | 0.767228380269585
      | 0.795433506084817
      | 0.826421878857641
      | 0.861000000000000
      | 0.899672183478468
      | 0.941733993478140
      | 0.986178806738742
      | 1.03200000000000
      | 1.07844226081654
      | 1.12575552000262
      | 1.17444101918739
      | 1.22500000000000
      | 1.27765252325536
      | 1.33149392651137
      | 1.38533836651170
      | 1.43800000000000
      | 1.48843202116203
      | 1.53614377395190
      | 1.58078363976582
      | 1.62200000000000
      | 1.65933814209653
      | 1.69193097768103
      | 1.71880832442502
      | 1.73900000000000
      | 1.75165291045186
      | 1.75638231532399
      | 1.75292056253412
      | 1.74100000000000
      | 1.72026896609601
      | 1.69003976102303
      | 1.64954067543852
      | 1.59800000000000
      | 1.53500560016408
      | 1.46158364058391
      | 1.37911986071179
      | 1.28900000000000
      | 1.19256800824768
      | 1.09100067664133
      | 0.985433006714323
      | 0.877000000000000
      | 0.767175491845209
      | 0.658788652850752
      | 0.555007487430919
      | 0.459000000000000
      | 0.373308149371486
      | 0.297969711955659
      | 0.232396418562003
      | 0.176000000000000
      | 0.128170035668849
      | 0.0882074993266129
      | 0.0553912133210702
      | 0.0290000000000000
      | 0.00830858295311821
      | -0.00742470926211037
      | -0.0189456468462838
      | -0.0270000000000000
      | -0.0322793674813219
      | -0.0352586622781714
      | -0.0363586259359352
      | -0.0360000000000000
      | -0.0345973630278306
      | -0.0325406416252041
      | -0.0302135994099755
      | -0.0280000000000000
      | -0.0261905554073556
      | -0.0247037712210123
      | -0.0233651014241628
      | -0.0220000000000000
      | -0.0204841653427468
      | -0.0188942734907467
      | -0.0173572448933732
      | -0.0160000000000000
      | -0.0149196582216572
      | -0.0140941348160010
      | -0.0134715440023443
      | -0.0130000000000000
      | -0.0126340767706245
      | -0.0123541872452493
      | -0.0121472040972494
      | -0.0120000000000000
      | -0.0119034096958447
      | -0.0118641162030018
      | -0.0118927646086579
      | -0.0120000000000000
      | -0.0121897844459966
      | -0.0124393479427436
      | -0.0127192374681188
      | -0.0130000000000000
      | -0.0132593275201690
      | -0.0135034920260239
      | -0.0137459105188668
      | -0.0140000000000000
      | -0.0142729054733275
      | -0.0145466839531609
      | -0.0147971204564139
      | -0.0150000000000000
      | -0.0151334255865212
      | -0.0151847721613325
      | -0.0151437326554777
      | -0.0150000000000000
      | -0.0147402671805879
      | -0.0143392274015089
      | -0.0137685739216755
      | -0.0130000000000000
      | -0.0120148806911273
      | -0.0108333182326318
      | -0.00948509665782044
      | -0.00800000000000000
      | -0.00640333505490292
      | -0.00470249966796380
      | -0.00290041444704278
      | -0.00100000000000000
      | 0.000987595910738992
      | 0.00301831690448703
      | 0.00503987944599156
      | 0.00700000000000000
      | 0.00884357641194696
      | 0.0105042320500157
      | 0.0119127716630766
      | 0.0130000000000000
      | 0.0137162234414732
      | 0.0140897548954503
      | 0.0141684089017022
      | 0.0140000000000000
      | 0.0136196548221603
      | 0.0130117483681832
      | 0.0121479677301145
      | 0.0110000000000000
      | 0.00953953226988547
      | 0.00773825163181676
      | 0.00556784517783966
      | 0.00300000000000000]
  des_hip_torque [Nm] : Outport
  wires:
  body_weigth [Kg]/1 -> Product/2
  assistance_level [%]/1 -> Gain/1
  Gain/1 -> Product/3
  stride %/1 -> Sum/1
  shift %/1 -> Sum/2
  winterAnkleFastSmooth/1 -> Embedded MATLAB Function/1(T)
  Embedded MATLAB Function/1(Tout) -> Product/1
  gain_pos/1 -> Embedded MATLAB Function/2(gain_pos)
  gain_neg/1 -> Embedded MATLAB Function/3(gain_neg)
  Sum/1 -> Gain1/1
  Product/1 -> des_hip_torque [Nm]/1
  Gain1/1 -> winterAnkleFastSmooth/1

== system AFO_Assistance/HIGH LEVEL CONTROL (200 Hz)/HIP_assistive_controller/stride % calculation ==
  step_trigger : Inport
  timer : Inport  Port=2
  step_freq_estimated : Inport  Port=3
  Product1 : Product  RndMeth=Zero
  Sum : Sum  Inputs=|-+
  take step start and period : Subsystem  TreatAsAtomicUnit=on
  to% : Gain  Gain=100  SampleTime=0.01
  step_start [s] : Outport
  freq_in_step [Hz] : Outport  Port=2
  stride % : Outport  Port=3
  wires:
  Product1/1 -> to%/1
  Sum/1 -> Product1/1
  take step start and period/2(frequency for the step) -> freq_in_step [Hz]/1
  step_freq_estimated/1 -> take step start and period/2(actual;_frequency), Product1/2
  take step start and period/1(time_count_stepon) -> Sum/1, step_start [s]/1
  timer/1 -> Sum/2, take step start and period/1(time_counter)
  step_trigger/1 -> take step start and period/Trigger
  to%/1 -> stride %/1

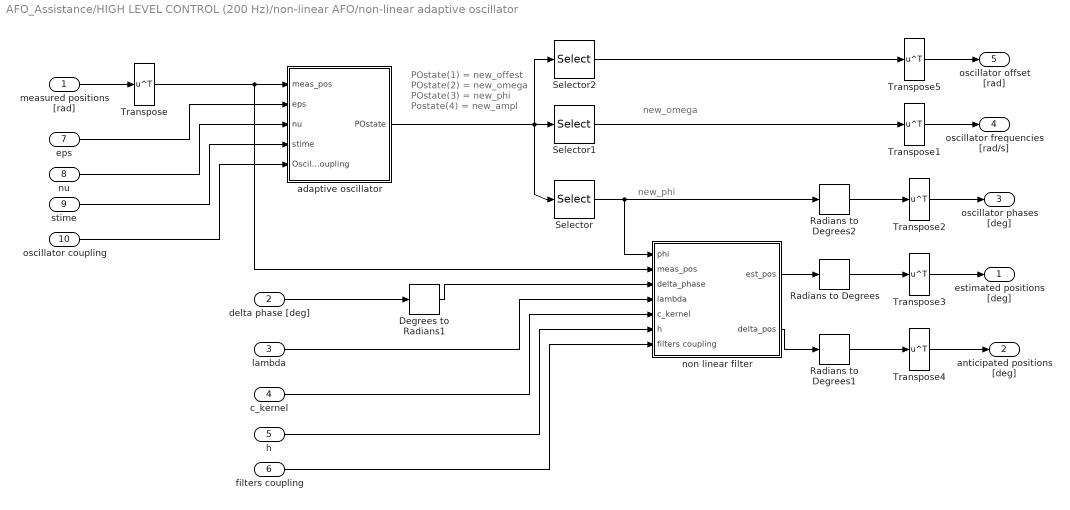
== system AFO_Assistance/HIGH LEVEL CONTROL (200 Hz)/non-linear AFO/non-linear adaptive oscillator ==
  note: POstate(1) = new_offest
      | POstate(2) = new_omega
      | POstate(3) = new_phi
      | Postate(4) = new_ampl
  note: new_omega
  note: new_phi
  measured positions [rad] : Inport
  delta phase [deg] : Inport  Port=2
  lambda : Inport  Port=3
  c_kernel : Inport  Port=4
  h : Inport  Port=5
  filters coupling : Inport  Port=6
  eps : Inport  Port=7
  nu : Inport  Port=8
  stime : Inport  Port=9
  oscillator coupling : Inport  Port=10
  Degrees to Radians1 : simulink_extras/Transformations/Degrees to Radians
  Radians to Degrees : simulink_extras/Transformations/Radians to Degrees
  Radians to Degrees1 : simulink_extras/Transformations/Radians to Degrees
  Radians to Degrees2 : simulink_extras/Transformations/Radians to Degrees
  Selector : Selector  NumberOfDimensions=2  InputPortWidth=3  IndexOptions=Index vector (dialog),Index vector (dialog)  Indices=3,1:4  OutputSizes=1,1
  Selector1 : Selector  NumberOfDimensions=2  InputPortWidth=3  IndexOptions=Index vector (dialog),Index vector (dialog)  Indices=2,1:4  OutputSizes=1,1
  Selector2 : Selector  NumberOfDimensions=2  InputPortWidth=3  IndexOptions=Index vector (dialog),Index vector (dialog)  Indices=1,1:4  OutputSizes=1,1
  Transpose{,1..5} (6 alike) : Math  Operator=transpose
  adaptive oscillator : Subsystem
  non linear filter : Subsystem
  estimated positions [deg] : Outport
  anticipated positions [deg] : Outport  Port=2
  oscillator phases [deg] : Outport  Port=3
  oscillator frequencies [rad/s] : Outport  Port=4
  oscillator offset [rad] : Outport  Port=5
  wires:
  adaptive oscillator/1(POstate) -> Selector/1, Selector1/1, Selector2/1
  Selector/1 -> non linear filter/1(phi), Radians to Degrees2/1
  non linear filter/1(est_pos) -> Radians to Degrees/1
  non linear filter/2(delta_pos) -> Radians to Degrees1/1
  measured positions [rad]/1 -> Transpose/1
  Radians to Degrees/1 -> Transpose3/1
  Radians to Degrees1/1 -> Transpose4/1
  Radians to Degrees2/1 -> Transpose2/1
  Selector1/1 -> Transpose1/1
  Transpose/1 -> adaptive oscillator/1(meas_pos), non linear filter/2(meas_pos)
  Transpose4/1 -> anticipated positions [deg]/1
  Transpose3/1 -> estimated positions [deg]/1
  Transpose2/1 -> oscillator phases [deg]/1
  Transpose1/1 -> oscillator frequencies [rad/s]/1
  delta phase [deg]/1 -> Degrees to Radians1/1
  Degrees to Radians1/1 -> non linear filter/3(delta_phase)
  lambda/1 -> non linear filter/4(lambda)
  c_kernel/1 -> non linear filter/5(c_kernel)
  h/1 -> non linear filter/6(h)
  filters coupling/1 -> non linear filter/7(filters coupling)
  eps/1 -> adaptive oscillator/2(eps)
  nu/1 -> adaptive oscillator/3(nu)
  stime/1 -> adaptive oscillator/4(stime)
  oscillator coupling/1 -> adaptive oscillator/5(Oscillator coupling)
  Transpose5/1 -> oscillator offset [rad]/1
  Selector2/1 -> Transpose5/1

== system AFO_Assistance/HIGH LEVEL CONTROL (200 Hz)/HIP_assistive_controller/stride % calculation/take step start and period ==
  time_counter : Inport
  actual;_frequency : Inport  Port=2
  Trigger : TriggerPort  VariantControl=(inherit)
  time_count_stepon : Outport
  frequency for the step : Outport  Port=2
  wires:
  actual;_frequency/1 -> frequency for the step/1
  time_counter/1 -> time_count_stepon/1

== system AFO_Assistance/HIGH LEVEL CONTROL (200 Hz)/non-linear AFO/non-linear adaptive oscillator/adaptive oscillator ==
  note: 0: no coupling
      | 1: hip coupled
      | 2: knee coupled
      | 3: hip and knee coupled
      | 4: right and left coupled
      | 5: all to all coupled
  note: POstate(1) = new_offest
      | POstate(2) = new_omega
      | POstate(3) = new_phi
      | Postate(4) = new_ampl
  note: eps = 6
      | nu = 0.25
      | stime = 0.001
  meas_pos : Inport
  eps : Inport  Port=2
  nu : Inport  Port=3
  stime : Inport  Port=4
  Oscillator coupling : Inport  Port=5
  Embedded MATLAB Function : MATLAB Function  TreatAsAtomicUnit=on
  Mux : Mux  Inputs=3
  Unit Delay : UnitDelay  InitialCondition=repmat([0;pi/4;ones(6,1)*pi/2;ones(6,1)*0],1,4)  SampleTime=-1
  POstate : Outport
  wires:
  meas_pos/1 -> Embedded MATLAB Function/1(meas_pos)
  Embedded MATLAB Function/1(POstate_out) -> POstate/1, Unit Delay/1
  Unit Delay/1 -> Embedded MATLAB Function/4(POstate_in)
  Oscillator coupling/1 -> Embedded MATLAB Function/3(coupling)
  Mux/1 -> Embedded MATLAB Function/2(parameters)
  eps/1 -> Mux/1
  nu/1 -> Mux/2
  stime/1 -> Mux/3

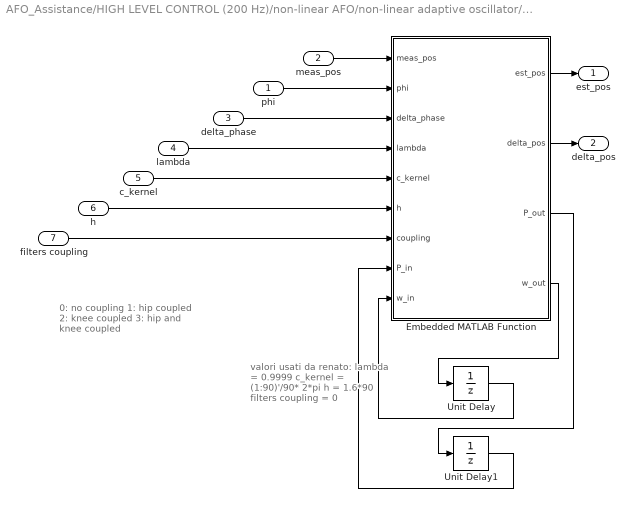
== system AFO_Assistance/HIGH LEVEL CONTROL (200 Hz)/non-linear AFO/non-linear adaptive oscillator/non linear filter ==
  note: 0: no coupling
      | 1: hip coupled
      | 2: knee coupled
      | 3: hip and knee coupled
  note: valori usati da renato:
      | lambda = 0.9999
      | c_kernel = (1:90)'/90* 2*pi
      | h = 1.6*90
      | filters coupling = 0
  phi : Inport
  meas_pos : Inport  Port=2
  delta_phase : Inport  Port=3
  lambda : Inport  Port=4
  c_kernel : Inport  Port=5
  h : Inport  Port=6
  filters coupling : Inport  Port=7
  Embedded MATLAB Function : MATLAB Function  TreatAsAtomicUnit=on
  Unit Delay : UnitDelay  InitialCondition=zeros(90,4)  SampleTime=-1
  Unit Delay1 : UnitDelay  InitialCondition=ones(90,4)  SampleTime=-1
  est_pos : Outport
  delta_pos : Outport  Port=2
  wires:
  Embedded MATLAB Function/4(w_out) -> Unit Delay/1
  Unit Delay/1 -> Embedded MATLAB Function/9(w_in)
  Embedded MATLAB Function/3(P_out) -> Unit Delay1/1
  Unit Delay1/1 -> Embedded MATLAB Function/8(P_in)
  meas_pos/1 -> Embedded MATLAB Function/1(meas_pos)
  phi/1 -> Embedded MATLAB Function/2(phi)
  delta_phase/1 -> Embedded MATLAB Function/3(delta_phase)
  filters coupling/1 -> Embedded MATLAB Function/7(coupling)
  Embedded MATLAB Function/1(est_pos) -> est_pos/1
  Embedded MATLAB Function/2(delta_pos) -> delta_pos/1
  lambda/1 -> Embedded MATLAB Function/4(lambda)
  c_kernel/1 -> Embedded MATLAB Function/5(c_kernel)
  h/1 -> Embedded MATLAB Function/6(h)

== stateflow chart AFO_Assistance/Motor Initialization/Motor Initliazation1 ==
  state inits
    entry:
    Motor_controlword = 0;
  note: The first commandword to the motor must be 0!
  state inits1
    entry:
    Motor_controlword = 6;
  state inits3
    entry:
    Motor_controlword = 128;
  note: If the model starts with the motor in Fault stat
      | this block will attempt to clear it
  state inits2
    entry:
    Motor_controlword = 15;
  (default) -> inits
  inits3 -> inits : [Stateword == 1632]
  inits -> (junction 12) [order 2]
  inits2 -> inits [order 2] : [Stateword == 999| Stateword == 64]
  inits1 -> inits [order 3] : [Stateword == 999 | Stateword == 64 ]
  inits -> inits1 [order 1] : [Stateword == 1632]
  inits1 -> (junction 12) [order 2]
  (junction 12) -> inits3 : [Stateword == 1576 |Stateword == 8]
  inits2 -> (junction 12) [order 1]
  inits1 -> inits2 [order 1] : [Stateword == 1569]
  data: Stateword input; Motor_controlword output

== matlab function AFO_Assistance/Subsystem6/MATLAB Function ==
  data: sig_in input; newbuf output; prev_buf input; N input; prev_updated_idx input; last_updated_idx output
function [newbuf,last_updated_idx]=circ_buffer(sig_in,prev_buf,N,prev_updated_idx)
    newbuf=prev_buf;
    last_updated_idx=next_idx(prev_updated_idx,N);
    newbuf(last_updated_idx)=sig_in;
end

function out=next_idx(t,N)
out=mod(t,N)+1;
end

== matlab function AFO_Assistance/Subsystem6/MATLAB Function1 ==
  data: sig_in input; newbuf output; prev_buf input; N input; prev_updated_idx input; last_updated_idx output
function [newbuf,last_updated_idx]=circ_buffer(sig_in,prev_buf,N,prev_updated_idx)
    newbuf=prev_buf;
    last_updated_idx=next_idx(prev_updated_idx,N);
    newbuf(last_updated_idx)=sig_in;
end

function out=next_idx(t,N)
out=mod(t,N)+1;
end
